simulink model "sim1"  (Simulink 7.6)
settings: Solver=FixedStepDiscrete  StartTime=0.0  StopTime=3000  FixedStep=1  RelTol=1e-3
settings Model: Creator=jordan  LastModifiedBy=jordan
settings OptimizationCC: BlockReduction=off  ConditionallyExecuteInputs=off

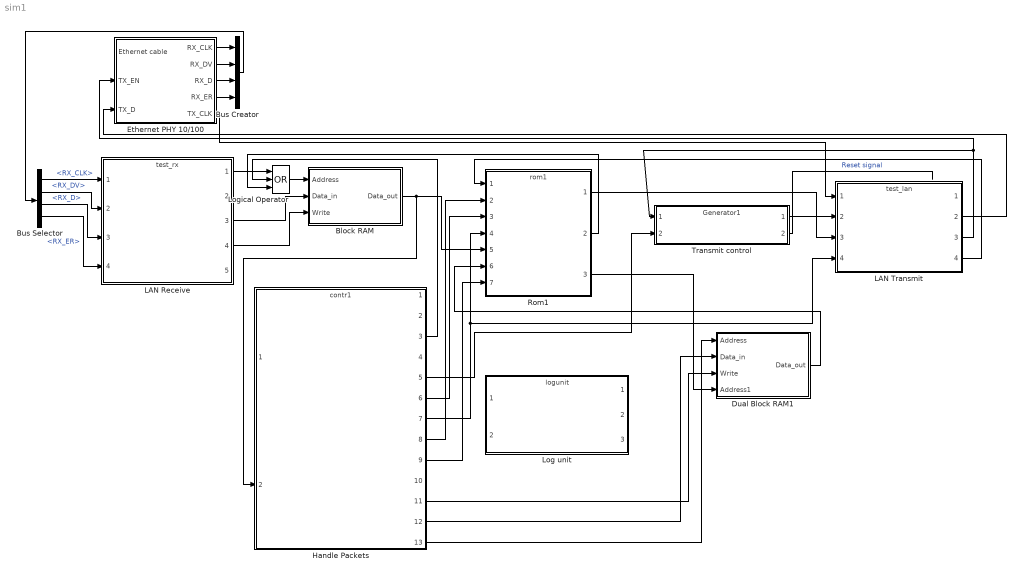
== system sim1 ==
  Block RAM : Subsystem
  Bus Creator : BusCreator  Inputs='RX_CLK','RX_DV','RX_D','RX_ER'
  Bus Selector : BusSelector  OutputSignals=RX_CLK,RX_DV,RX_D,RX_ER
  Dual Block RAM1 : Subsystem
  Ethernet PHY 10/100 : Subsystem
  Handle Packets : ModelReference  ModelNameDialog=contr1  SimulationMode=Normal  ModelReferenceVersion=1.464  CopyOfModelName=contr1
  LAN Receive : ModelReference  ModelNameDialog=test_rx  SimulationMode=Normal  ModelReferenceVersion=1.282  CopyOfModelName=test_rx
  LAN Transmit : ModelReference  ModelNameDialog=test_lan  SimulationMode=Normal  ModelReferenceVersion=1.198  CopyOfModelName=test_lan
  Log unit : ModelReference  ModelNameDialog=logunit  SimulationMode=Normal  ModelReferenceVersion=1.519  CopyOfModelName=logunit
  Logical Operator : Logic  Operator=OR  Inputs=3  AllPortsSameDT=off  OutDataTypeStr=boolean
  Rom1 : ModelReference  ModelNameDialog=rom1  SimulationMode=Normal  ModelReferenceVersion=1.163  CopyOfModelName=rom1
  Transmit control : ModelReference  ModelNameDialog=Generator1  SimulationMode=Normal  ModelReferenceVersion=1.104  CopyOfModelName=Generator1
  wires:
  Handle Packets/3 -> Logical Operator/2
  Block RAM/1(Data_out) -> Handle Packets/2, Rom1/5
  LAN Receive/3 -> Block RAM/2(Data_in)
  LAN Receive/4 -> Block RAM/3(Write)
  LAN Receive/1 -> Logical Operator/1
  Transmit control/1 -> LAN Transmit/2
  Transmit control/2 -> ?  "Reset signal"
  Handle Packets/5 -> Transmit control/2
  LAN Transmit/3 -> Transmit control/1, Ethernet PHY 10/100/2(TX_EN)
  Logical Operator/1 -> Block RAM/1(Address)
  Rom1/1 -> LAN Transmit/3
  LAN Transmit/4 -> Rom1/1
  Handle Packets/8 -> Rom1/2
  Handle Packets/7 -> LAN Transmit/4, Rom1/4
  Handle Packets/6 -> Rom1/3
  Rom1/2 -> Logical Operator/3
  Handle Packets/9 -> Rom1/7
  Ethernet PHY 10/100/1(RX_CLK) -> Bus Creator/1
  Ethernet PHY 10/100/2(RX_DV) -> Bus Creator/2
  Ethernet PHY 10/100/3(RX_D) -> Bus Creator/3
  Ethernet PHY 10/100/4(RX_ER) -> Bus Creator/4
  Bus Creator/1 -> Bus Selector/1
  Bus Selector/1 -> LAN Receive/1  "<RX_CLK>"
  Bus Selector/2 -> LAN Receive/2  "<RX_DV>"
  Bus Selector/3 -> LAN Receive/3  "<RX_D>"
  Bus Selector/4 -> LAN Receive/4  "<RX_ER>"
  LAN Transmit/2 -> Ethernet PHY 10/100/3(TX_D)
  Ethernet PHY 10/100/5(TX_CLK) -> LAN Transmit/1
  Dual Block RAM1/1(Data_out) -> Rom1/6
  Rom1/3 -> Dual Block RAM1/4(Address1)
  Handle Packets/13 -> Dual Block RAM1/1(Address)
  Handle Packets/12 -> Dual Block RAM1/2(Data_in)
  Handle Packets/11 -> Dual Block RAM1/3(Write)

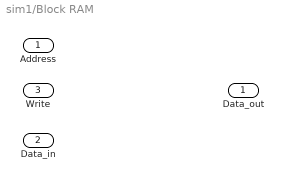
== system sim1/Block RAM ==
  Address : Inport  OutDataTypeStr=boolean
  Data_in : Inport  Port=2  OutDataTypeStr=boolean
  Write : Inport  Port=3  OutDataTypeStr=boolean
  Data_out : Outport

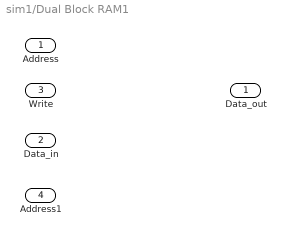
== system sim1/Dual Block RAM1 ==
  Address : Inport  OutDataTypeStr=boolean
  Data_in : Inport  Port=2  OutDataTypeStr=boolean
  Write : Inport  Port=3  OutDataTypeStr=boolean
  Address1 : Inport  Port=4  OutDataTypeStr=boolean
  Data_out : Outport

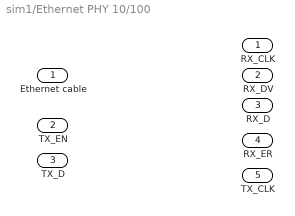
== system sim1/Ethernet PHY 10/100 ==
  Ethernet cable : Inport  OutDataTypeStr=boolean
  TX_EN : Inport  Port=2  OutDataTypeStr=boolean
  TX_D : Inport  Port=3  OutDataTypeStr=boolean
  RX_CLK : Outport
  RX_DV : Outport  Port=2
  RX_D : Outport  Port=3
  RX_ER : Outport  Port=4
  TX_CLK : Outport  Port=5
